simulink model "rotax_engine_model"  (R2026a)
settings: Solver=VariableStepAuto  StopTime=300
settings Model: Creator=GOD  LastModifiedBy=GOD

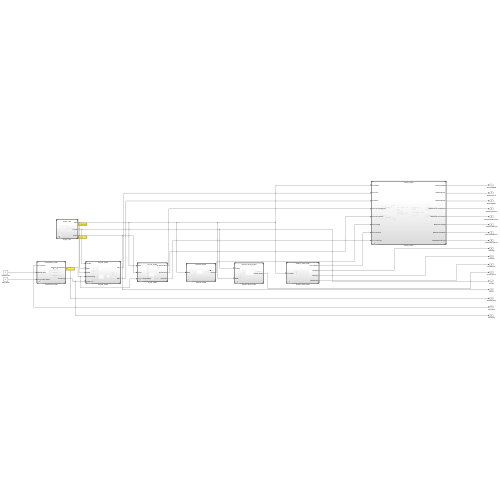
[thumbnail: Simulink's stored preview of the top-level diagram]
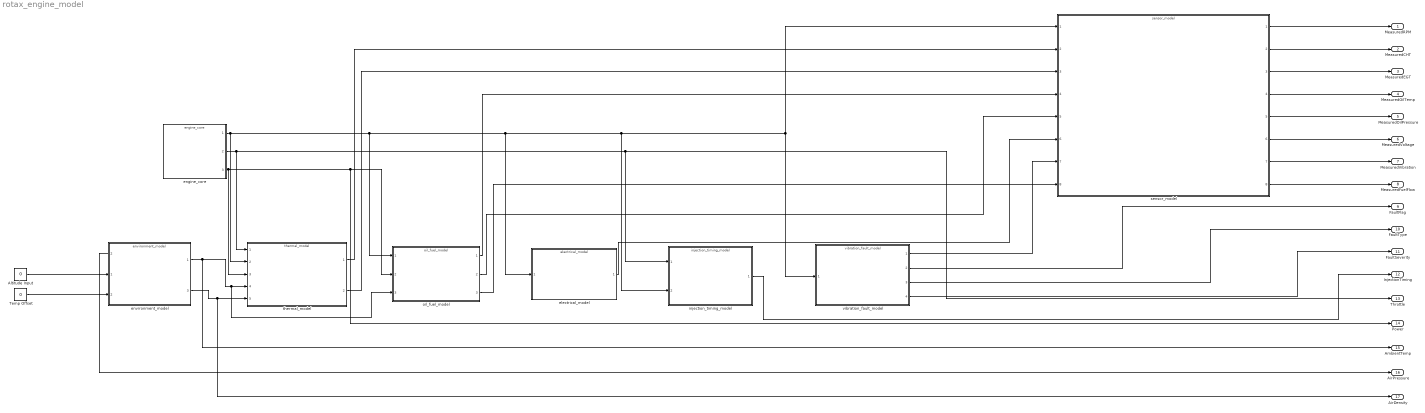
== system rotax_engine_model ==
  Altitude Input : Constant  Value=0
  Temp Offset : Constant  Value=0
  electrical_model : ModelReference  ModelNameDialog=electrical_model.slx  SimulationMode=Normal  ModelReferenceVersion=1.2
  engine_core : ModelReference  ModelNameDialog=engine_core.slx  SimulationMode=Normal  ModelReferenceVersion=1.10
  environment_model : ModelReference  ModelNameDialog=environment_model.slx  SimulationMode=Normal  ModelReferenceVersion=1.5
      settings: PortSchema="{\"entries\":[{\"content\":{\"sides\":[{\"content\":{\"connectorIds\":[\"Out2\",\"In1\",\"In2\"]},\"type\":\"ConnectorPlacement.EquallySpacedRectSide\",\"uuid\":\"93a5604f-b0be-433b-85bd-421dd1e3d138\"},{\"content\":{\"connectorIds\":[\"Out1\",\"Out3\"],\"side\":\"RIGHT\"},\"type\":\"ConnectorPlacement.EquallySpacedRectSide\",\"uuid\":\"8ef1e0b5-0d11-42ea-9474-27754fd8dcbe\"},{\"content\":{\"side\":\"TOP\"},\"type\":\"ConnectorPlacement.EquallySpacedRectSide\",\"uuid\":\"03ccf673-eb8a-44b8-bbce-76c277eb4791\"}]},\"type\":\"ConnectorPlacement.EquallySpacedConnector\",\"uuid\":\"3e9d8c6f-6482-451c-a2c1-4f18d454d8f1\"}],\"packageUris\":[\"http://schema.mathworks.com/mf0/Connector/R2020b\"],\"version\":\"1.0\"}"
  injection_timing_model : ModelReference  ModelNameDialog=injection_timing_model.slx  SimulationMode=Normal  ModelReferenceVersion=1.2
  oil_fuel_model : ModelReference  ModelNameDialog=oil_fuel_model.slx  SimulationMode=Normal  ModelReferenceVersion=1.5
  sensor_model : ModelReference  ModelNameDialog=sensor_model.slx  SimulationMode=Normal  ModelReferenceVersion=1.7
  thermal_model : ModelReference  ModelNameDialog=thermal_model.slx  SimulationMode=Normal  ModelReferenceVersion=1.6
  vibration_fault_model : ModelReference  ModelNameDialog=vibration_fault_model.slx  SimulationMode=Normal  ModelReferenceVersion=1.8
  MeasuredRPM : Outport
  MeasuredCHT : Outport  Port=2
  MeasuredEGT : Outport  Port=3
  MeasuredOilTemp : Outport  Port=4
  MeasuredOilPressure : Outport  Port=5
  MeasuredVoltage : Outport  Port=6
  MeasuredVibration : Outport  Port=7
  MeasuredFuelFlow : Outport  Port=8
  FaultFlag : Outport  Port=9
  FaultType : Outport  Port=10
  FaultSeverity : Outport  Port=11
  InjectionTiming : Outport  Port=12
  Throttle : Outport  Port=13
  Power : Outport  Port=14
  AmbientTemp : Outport  Port=15
  AirPressure : Outport  Port=16
  AirDensity : Outport  Port=17
  wires:
  Altitude Input/1 -> environment_model/1
  Temp Offset/1 -> environment_model/2
  environment_model/1 -> AmbientTemp/1, oil_fuel_model/3, thermal_model/4
  environment_model/3 -> AirDensity/1, thermal_model/5
  engine_core/2 -> Throttle/1, injection_timing_model/1, thermal_model/1
  engine_core/1 -> vibration_fault_model/1, sensor_model/1, injection_timing_model/2, electrical_model/1, oil_fuel_model/1, thermal_model/2
  engine_core/3 -> Power/1, oil_fuel_model/2, thermal_model/3
  thermal_model/1 -> sensor_model/2
  thermal_model/2 -> sensor_model/3
  oil_fuel_model/1 -> sensor_model/4
  oil_fuel_model/2 -> sensor_model/5
  electrical_model/1 -> sensor_model/6
  vibration_fault_model/1 -> sensor_model/7
  oil_fuel_model/3 -> sensor_model/8
  sensor_model/3 -> MeasuredEGT/1
  sensor_model/2 -> MeasuredCHT/1
  sensor_model/1 -> MeasuredRPM/1
  sensor_model/4 -> MeasuredOilTemp/1
  sensor_model/5 -> MeasuredOilPressure/1
  sensor_model/6 -> MeasuredVoltage/1
  sensor_model/7 -> MeasuredVibration/1
  sensor_model/8 -> MeasuredFuelFlow/1
  vibration_fault_model/2 -> FaultFlag/1
  vibration_fault_model/3 -> FaultType/1
  vibration_fault_model/4 -> FaultSeverity/1
  injection_timing_model/1 -> InjectionTiming/1
  environment_model/2 -> AirPressure/1
